simulink model "fANDgByFullMatlab"  (R2016b)
settings: Solver=FixedStepDiscrete  StartTime=0.0  StopTime=10.0  RelTol=1e-3
settings Model: DataTypeOverride=Off  Creator=hasee  LastModifiedBy=hasee
settings DataIOCC: LimitDataPoints=on  SaveOutput=off  SaveTime=off
settings OptimizationCC: BlockReduction=off  ConditionallyExecuteInputs=off  DefaultParameterBehavior=Inlined  LifeSpan=inf
settings DebuggingCC: AlgebraicLoopMsg=error  SingleTaskRateTransMsg=error  AllowSymbolicDim=off  StrictBusMsg=ErrorOnBusTreatedAsVector  SFUnexpectedBacktrackingDiag=warning  SFNoUnconditionalDefaultTransitionDiag=warning  SFExecutionAtInitializationDiag=none
settings HardwareCC: ProdBitPerPointer=32  ProdBitPerSizeT=32  ProdBitPerPtrDiffT=32  ProdLargestAtomicFloat=None  ProdIntDivRoundTo=Undefined  ProdEndianess=Unspecified  ProdWordSize=32  ProdHWDeviceType=ASIC/FPGA->ASIC/FPGA  ProdEqTarget=off
settings GRTTargetCC: TargetLangStandard=C89/C90 (ANSI)  GeneratePreprocessorConditionals=Disable all
settings ConfigComp: CovScope=ReferencedModels  CovMetricSettings=dw  CovHtmlReporting=on  CovSaveCumulativeToWorkspaceVar=on  CovSaveSingleToWorkspaceVar=on  CovExternalEMLEnable=off  CovSFcnEnable=off

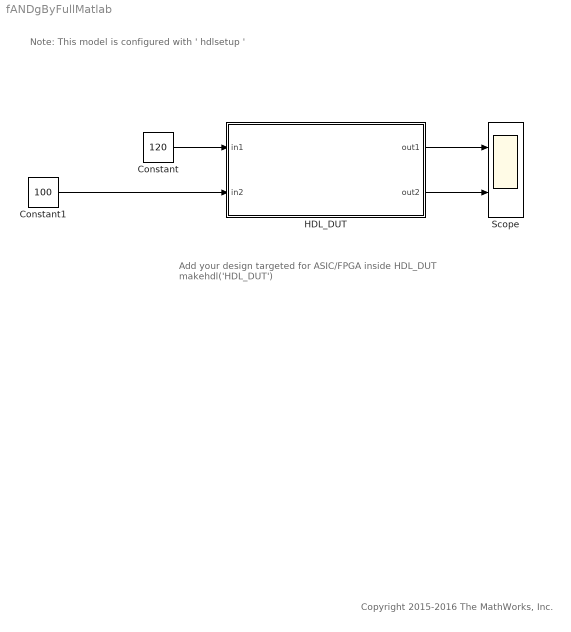
== system fANDgByFullMatlab ==
  note: Note: This model is configured with ' hdlsetup '
  note: Add your design targeted for ASIC/FPGA inside HDL_DUT
      | makehdl('HDL_DUT')
  note: Copyright 2015-2016 The MathWorks, Inc.
  Constant : Constant  Value=120  OutDataTypeStr=int8  SampleTime=-1
  Constant1 : Constant  Value=100  OutDataTypeStr=int8  SampleTime=-1
  HDL_DUT : Subsystem
  Scope : Scope  NumInputPorts=2
  wires:
  Constant/1 -> HDL_DUT/1(in1)
  Constant1/1 -> HDL_DUT/2(in2)
  HDL_DUT/1(out1) -> Scope/1
  HDL_DUT/2(out2) -> Scope/2

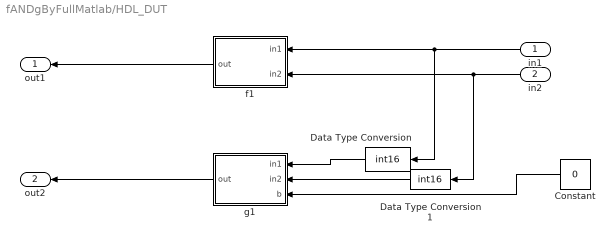
== system fANDgByFullMatlab/HDL_DUT ==
  in1 : Inport
  in2 : Inport  Port=2
  Constant : Constant  Value=0  OutDataTypeStr=boolean  SampleTime=-1
  Data Type Conversion : DataTypeConversion  OutDataTypeStr=int16
  Data Type Conversion1 : DataTypeConversion  OutDataTypeStr=int16
  f1 : MATLAB Function  TreatAsAtomicUnit=on
  g1 : MATLAB Function  TreatAsAtomicUnit=on
  out1 : Outport
  out2 : Outport  Port=2
  wires:
  in1/1 -> Data Type Conversion/1, f1/1(in1)
  in2/1 -> Data Type Conversion1/1, f1/2(in2)
  f1/1(out) -> out1/1
  Constant/1 -> g1/3(b)
  g1/1(out) -> out2/1
  Data Type Conversion/1 -> g1/1(in1)
  Data Type Conversion1/1 -> g1/2(in2)

== matlab function fANDgByFullMatlab/HDL_DUT/g1 ==
  data: in1 input; out output; in2 input; b input
function out = fcn(in1, in2, b)
%#codegen
if (b == 0)
    out=in1 + in2;
else
    out=-in1 + in2;
end

== matlab function fANDgByFullMatlab/HDL_DUT/f1 ==
  data: in1 input; out output; in2 input
function out = fcn(in1, in2)
%#codegen
if (in1>0 && in2>0) ||(in1<0 && in2<0)
    out=min(abs(in1),abs(in2));
else
    out=-min(abs(in1),abs(in2));
end
